simulink model "UberSpurs"  (R2015b)
settings: Solver=VariableStepAuto  StartTime=0.0  StopTime=5000  RelTol=1e-3
libraries: simulink x54
(part 6 of 6)

== stateflow chart UberSpurs/baggerAssignmentControl_roundRobin ==
  state NotMultiScript
    (history)
    state AssignBagger1
      entry:
      baggerAssignment = 1;
    state AssignBagger3
      entry:
      baggerAssignment = 3;
    state AssignBagger2
      entry:
      baggerAssignment = 2;
    (default) -> AssignBagger1
    AssignBagger3 -> AssignBagger1 [order 1] : [bagger1Pause == 0]
    AssignBagger1 -> AssignBagger3 [order 2]
    AssignBagger1 -> AssignBagger2 [order 1] : [bagger2Pause == 0]
    AssignBagger2 -> AssignBagger1 [order 2] : [bagger3Pause == 1]
    AssignBagger3 -> AssignBagger2 [order 2]
    AssignBagger2 -> AssignBagger3 [order 1] : [bagger3Pause == 0]
  (default) -> (junction 3)
  (junction 3) -> NotMultiScript [order 2]
  (junction 3) -> (junction 10) [order 1] : [baggerAssignmentIN ==4]
      | {baggerAssignment =4;}
  NotMultiScript -> (junction 10)
  data: baggerAssignment output; bagger1Queue input; bagger1Pause input; bagger2Queue input; bagger2Pause input; bagger3Queue input; bagger3Pause input; baggerAssignmentIN input

== stateflow chart UberSpurs/baggerAssignmentControl_shortestQueue ==
  (junction 3) -> (junction 20) [order 3]
  (default) -> (junction 3)
  (junction 3) -> (junction 15) [order 2] : [bagger1Queue <= bagger2Queue & bagger1Queue <= bagger3Queue]
  (junction 15) -> (junction 20) [order 2] : [bagger1Queue > bagger2Queue]
  (junction 20) -> (junction 26) [order 1] : [bagger2Queue > bagger3Queue]
  (junction 20) -> (junction 26) [order 3] : [bagger2Pause == 1]
  (junction 15) -> (junction 20) [order 3] : [bagger1Pause ==1]
  (junction 3) -> (junction 10) [order 1] : [baggerAssignmentIN ==4]
      | {baggerAssignment =4;}
  (junction 15) -> (junction 17) [order 1] : [bagger1Pause ==0]
      | {baggerAssignment = 1;}
  (junction 20) -> (junction 23) [order 2] : [bagger2Pause == 0]
      | {baggerAssignment = 2;}
  (junction 26) -> (junction 30) : {baggerAssignment =3;}
  (junction 17) -> (junction 10)
  (junction 23) -> (junction 17)
  (junction 30) -> (junction 23)
  data: baggerAssignment output; bagger1Queue input; bagger1Pause input; bagger2Queue input; bagger2Pause input; bagger3Queue input; bagger3Pause input; baggerAssignmentIN input
